simulink model "slexFPGAPredictFixedPointExample"  (R2023b)
settings: Solver=FixedStepDiscrete  StartTime=0.0  StopTime=timeVector(end)  FixedStep=stepSize  RelTol=1e-3
undefined symbols (not defined in the file): X_MAX, X_MIN
libraries: statsLibrary x1
settings Model: DataTypeOverride=Off  MinMaxOverflowLogging=ForceOff  FPTShortcutValueString='{{},{''BaselineRun'',1,1,1,''BaselineRun'','''',{},''M'','''',''''},{''EmbeddedRun'',1,1,1,''EmbeddedRun'','''',{},''M'','''',''''},{''EmbeddedRun_2'',1,1,1,''EmbeddedRun_2'','''',{},''M'','''',''''},{''EmbeddedRun_3'',1,1,1,''EmbeddedRun_3'','''',{},''M'','''',''''},{''EmbeddedRun_4'',1,1,1,''EmbeddedRun_4'','''',{},''M'','''',''''},{''EmbeddedRun_5'',1,1,1,''EmbeddedRun_5'','''',{},''M'','''',''''},{''EmbeddedRun_6'',1,1,1,''EmbeddedRun_6'','''',{},''M'','''',''''}}'  SimulationMode=accelerator  Creator=The MathWorks, Inc.  LastModifiedBy=The MathWorks, Inc.
settings DataIOCC: SaveTime=off
settings OptimizationCC: BlockReduction=off  ConditionallyExecuteInputs=off  DefaultParameterBehavior=Inlined  InheritOutputTypeSmallerThanSingle=on
settings DebuggingCC: SignalRangeChecking=error  AlgebraicLoopMsg=error  InheritedTsInSrcMsg=none  SingleTaskRateTransMsg=error  IntegerOverflowMsg=none  ParameterDowncastMsg=none  ParameterOverflowMsg=none  ParameterPrecisionLossMsg=none  IntegerSaturationMsg=none
settings HardwareCC: ProdBitPerPointer=32  ProdBitPerSizeT=32  ProdBitPerPtrDiffT=32  ProdLargestAtomicFloat=None  ProdIntDivRoundTo=Undefined  ProdEndianess=Unspecified  ProdWordSize=32  ProdHWDeviceType=ASIC/FPGA->ASIC/FPGA  TargetBitPerLong=64  TargetBitPerPointer=64  TargetBitPerSizeT=64  TargetBitPerPtrDiffT=64  TargetLongLongMode=on  TargetIntDivRoundTo=Zero  TargetEndianess=LittleEndian  TargetWordSize=64  TargetHWDeviceType=Custom Processor->MATLAB Host Computer  ProdEqTarget=off
settings ModelReferenceCC: EnableRefExpFcnMdlSchedulingChecks=on

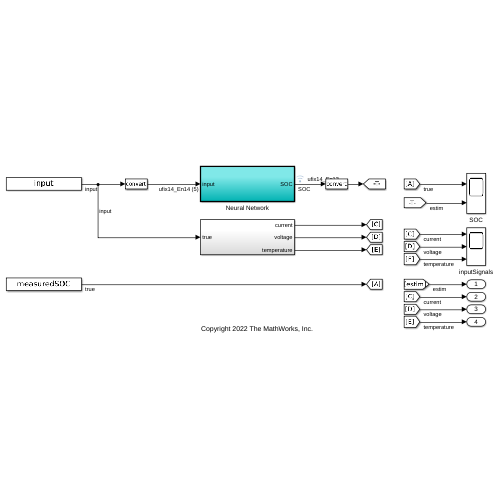
[thumbnail: Simulink's stored preview of the top-level diagram]
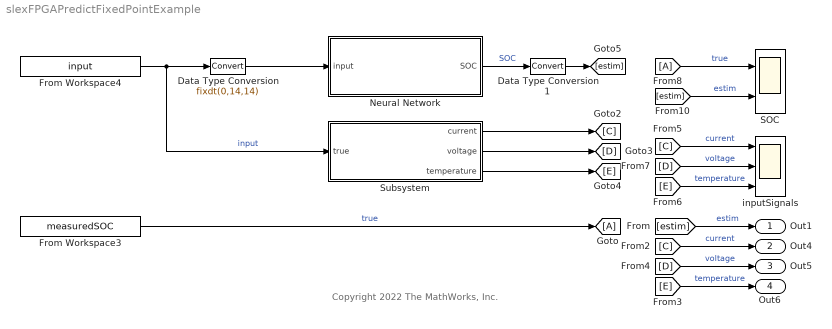
== system slexFPGAPredictFixedPointExample ==
  note: Copyright 2022 The MathWorks, Inc.
  Data Type Conversion : DataTypeConversion  OutDataTypeStr=fixdt(0,14,14)  SaturateOnIntegerOverflow=off  RndMeth=Floor
  Data Type Conversion1 : DataTypeConversion  SaturateOnIntegerOverflow=off  RndMeth=Floor
  From Workspace3 : FromWorkspace  VariableName=measuredSOC  SampleTime=-1
  From Workspace4 : FromWorkspace  VariableName=input  SampleTime=-1
  From8 : From
  Goto : Goto
  Neural Network : Subsystem  TreatAsAtomicUnit=on
  SOC : Scope  NumInputPorts=2
  Subsystem : Subsystem
  inputSignals : Scope  NumInputPorts=3
  Out1 : Outport
  Out4 : Outport  Port=2
  Out5 : Outport  Port=3
  Out6 : Outport  Port=4
  wires:
  Data Type Conversion1/1 -> [estim]
  Data Type Conversion/1 -> Neural Network/1(input)
  From Workspace4/1 -> Data Type Conversion/1, Subsystem/1(true)  "input"
  [D] -> Out5/1  "voltage"
  [E] -> inputSignals/3  "temperature"
  [estim] -> SOC/2  "estim"
  From8/1 -> SOC/1  "true"
  [C] -> Out4/1  "current"
  [D] -> inputSignals/2  "voltage"
  [C] -> inputSignals/1  "current"
  From Workspace3/1 -> Goto/1  "true"
  Neural Network/1(SOC) -> Data Type Conversion1/1  "SOC"
  Subsystem/3(temperature) -> [E]
  [estim] -> Out1/1  "estim"
  Subsystem/1(current) -> [C]
  Subsystem/2(voltage) -> [D]
  [E] -> Out6/1  "temperature"

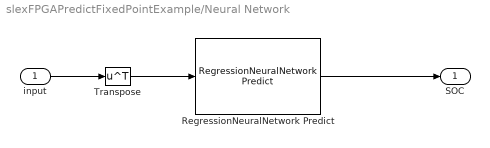
== system slexFPGAPredictFixedPointExample/Neural Network ==
  input : Inport  OutDataTypeStr=fixdt(0,14,14)  PortDimensions=[5]  SampleTime=10
  RegressionNeuralNetwork Predict : statsLibrary/Regression/RegressionNeuralNetwork Predict  TrainedLearner=nnetMdl  OutDataTypeStr=fixdt(0,14,13)  OutMin=[]  OutMax=[]  OutputLayerDataTypeStr=fixdt(1,14,12)  OutputLayerOutMin=[]  OutputLayerOutMax=[]  OutputLayerAdditionDataTypeStr=fixdt(0,14,13)  OutputLayerAdditionOutMin=[]  OutputLayerAdditionOutMax=[]  LayerSelector=Layer 1  Layer1DataTypeStr=fixdt(1,13,10)  Layer1OutMin=[]  Layer1OutMax=[]  Layer1AdditionDataTypeStr=fixdt(1,14,11)  Layer1AdditionOutMin=[]  Layer1AdditionOutMax=[]  Layer2DataTypeStr=fixdt(1,14,11)  Layer2OutMin=[]  Layer2OutMax=[]  Layer2AdditionDataTypeStr=fixdt(1,14,10)  Layer2AdditionOutMin=[]  Layer2AdditionOutMax=[]  Layer3OutMin=[]  Layer3OutMax=[]  Layer3AdditionOutMin=[]  Layer3AdditionOutMax=[]  Layer4OutMin=[]  Layer4OutMax=[]  Layer4AdditionOutMin=[]  Layer4AdditionOutMax=[]  Layer5OutMin=[]  Layer5OutMax=[]  Layer5AdditionOutMin=[]  Layer5AdditionOutMax=[]  Layer6OutMin=[]  Layer6OutMax=[]  Layer6AdditionOutMin=[]  Layer6AdditionOutMax=[]  Layer7OutMin=[]  Layer7OutMax=[]  Layer7AdditionOutMin=[]  Layer7AdditionOutMax=[]  Layer8OutMin=[]  Layer8OutMax=[]  Layer8AdditionOutMin=[]  Layer8AdditionOutMax=[]  Layer9OutMin=[]  Layer9OutMax=[]  Layer9AdditionOutMin=[]  Layer9AdditionOutMax=[]  Layer10OutMin=[]  Layer10OutMax=[]  Layer10AdditionOutMin=[]  Layer10AdditionOutMax=[]  Layer11OutMin=[]  Layer11OutMax=[]  Layer11AdditionOutMin=[]  Layer11AdditionOutMax=[]  StandardizedInputDataTypeStr=fixdt(1,12,8)  StandardizedInputOutMin=[]  StandardizedInputOutMax=[]  NumHiddenLayers=1
  Transpose : Math  Operator=transpose  OutDataTypeStr=double
  SOC : Outport  OutDataTypeStr=fixdt(0,14,13)  SampleTime=10
  wires:
  input/1 -> Transpose/1
  RegressionNeuralNetwork Predict/1 -> SOC/1
  Transpose/1 -> RegressionNeuralNetwork Predict/1

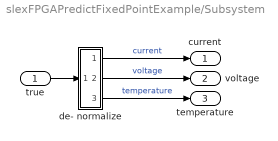
== system slexFPGAPredictFixedPointExample/Subsystem ==
  true : Inport
  de- normalize : Subsystem
  current : Outport
  voltage : Outport  Port=2
  temperature : Outport  Port=3
  wires:
  true/1 -> de- normalize/1(u)
  de- normalize/3(T) -> temperature/1  "temperature"
  de- normalize/1(I) -> current/1  "current"
  de- normalize/2(V) -> voltage/1  "voltage"

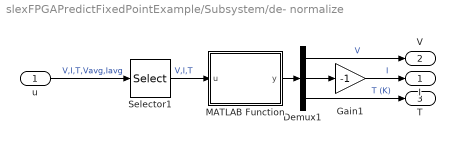
== system slexFPGAPredictFixedPointExample/Subsystem/de- normalize ==
  u : Inport
  Demux1 : Demux  Outputs=3
  Gain1 : Gain  Gain=-1
  MATLAB Function : MATLAB Function  TreatAsAtomicUnit=on
  Selector1 : Selector  InputPortWidth=5  IndexOptions=Index vector (dialog)  Indices=[1 2 3]  OutputSizes=1
  I : Outport
  V : Outport  Port=2
  T : Outport  Port=3
  wires:
  Gain1/1 -> I/1  "I"
  Selector1/1 -> MATLAB Function/1(u)  "V,I,T"
  Demux1/2 -> Gain1/1
  Demux1/1 -> V/1  "V"
  Demux1/3 -> T/1  "T (K)"
  MATLAB Function/1(y) -> Demux1/1
  u/1 -> Selector1/1  "V,I,T,Vavg,Iavg"

== matlab function slexFPGAPredictFixedPointExample/Subsystem/de- normalize/MATLAB Function ==
  data: u input; y output; X_MAX parameter; X_MIN parameter
function y = fcn(u, X_MAX, X_MIN)
y = (X_MAX-X_MIN).*u+X_MIN;
y(3) = y(3) + 273.15; % convert to K
